simulink model "CONTROL_01"  (R2018b)
settings: Solver=FixedStepAuto  StartTime=0.0  StopTime=30  FixedStep=0.01  RelTol=1e-3
model workspace: external: MATLAB File D:\OneDrive\STUDY\RIC LAB\PROJECT 6DOF\CODE\CODE 6DOF\07_CONTROL\CONTROL_02\ROBOT_DataFile.m (data not in the file)
undefined symbols (not defined in the file or in its folder): smiData, X, Y, Z
libraries: sm_lib x35, nesl_utility x7
(part 1 of 185)
settings Model: Creator=TMP  LastModifiedBy=TMP
settings DataIOCC: SaveTime=off
settings DebuggingCC: AlgebraicLoopMsg=none

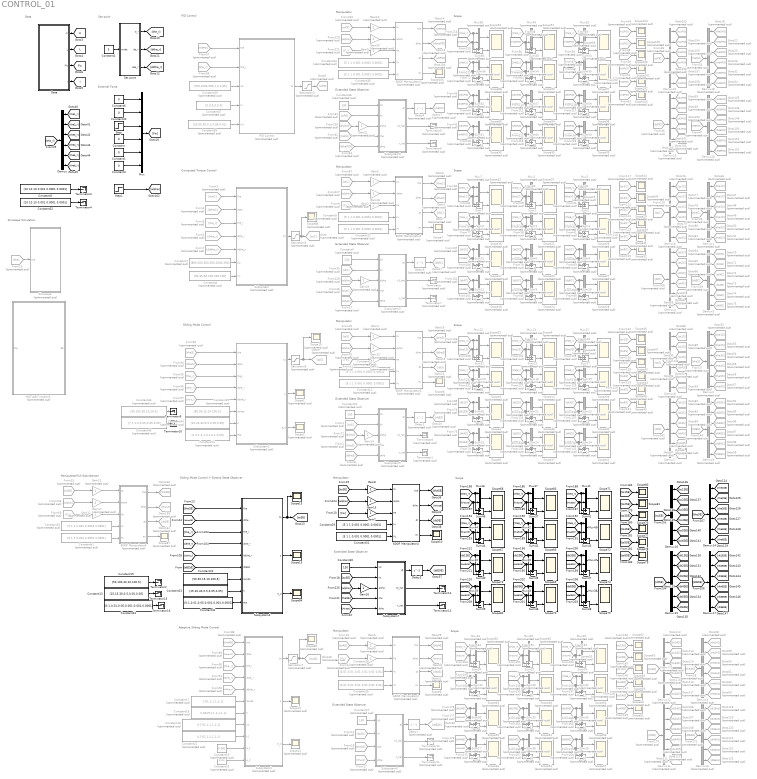
== system CONTROL_01 ==
  note: Extended State Observer
  note: Set point
  note: Simscape Simulation
  note: Data
  note: External Force
  note: Computed Torque Control
  note: Manipulator
  note: Sliding Mode Control
  note: Adaptive Sliding Mode Control
  note: Sliding Mode Control + Extend State Observer
  note: Extended State Observer
  note: Manipulator
  note: Extended State Observer
  note: Manipulator
  note: Extended State Observer
  note: Manipulator
  note: Scope
  note: Scope
  note: Scope
  note: Scope
  note: Extended State Observer
  note: PID Control
  note: Manipulator
  note: Scope
  note: Manipulator(full disturbance)
  6DOF Manipulator1 : Subsystem  Commented=on
  6DOF Manipulator2 : Subsystem  Commented=on
  6DOF Manipulator3 : Subsystem  Commented=on
  6DOF Manipulator4 : Subsystem
  6DOF Manipulator5 : Subsystem  Commented=on
  6DOF Manipulator6 : Subsystem  Commented=on
  Constant{,1,3,6,40} (5 alike) : Constant  Value=0
  Constant{9..12,33..35,41} (8 alike) : Constant  Commented=on  Value=[5 1 1 0.001 0.0001 0.0001]
  Constant13 : Constant  Value=[15,15,30,0.5,0.05,0.05]
  Constant14 : Constant  Commented=on  Value=[1.5,1.2,1,0.1,0.1,0.05]
  Constant15 : Constant  Value=[50,100,30,10,100,5]
  Constant16 : Constant  Commented=on  Value=0.001*[1,1,1,1,1,1]
  Constant17 : Constant  Commented=on  Value=1*[1,1,1,1,1,1]
  Constant18 : Constant  Commented=on  Value=0.1*[1,1,1,1,1,1]
  Constant19 : Constant  Commented=on  Value=0.001
  Constant2 : Constant  Value=3
  Constant20 : Constant  Commented=on  Value=0.01
  Constant21 : Constant  Commented=on  Value=0.1*[1,1,1,1,1,1]
  Constant22 : Constant  Commented=on  Value=130
  Constant23 : Constant  Value=[15,20,30,0.5,0.05,0.05]
  Constant24 : Constant  Value=[50,50,15,10,100,5]
  Constant25 : Constant  Commented=on  Value=[50,50,15,10,100,5]
  Constant26 : Constant  Commented=on  Value=[0.01 0.01 0.01 0.01 0.01 0.01]
  Constant27 : Constant  Commented=on  Value=100
  Constant28 : Constant  Commented=on  Value=[0.01 0.01 0.01 0.01 0.01 0.01]
  Constant29 : Constant  Value=[5 1 1 0.001 0.0001 0.0001]
  Constant30 : Constant  Value=130
  Constant31 : Constant  Value=[5 1 1 0.001 0.0001 0.0001]
  Constant32 : Constant  Value=[10 10 10 0.001 0.0001 0.0001]
  Constant36 : Constant  Commented=on  Value=130
  Constant37 : Constant  Commented=on  Value=[0,0,0,0,0,0]
  Constant38 : Constant  Commented=on  Value=[20,50,30,0.1,0.06,0.01]
  Constant39 : Constant  Commented=on  Value=[700,1200,500,1,2,0.05]
  Constant4 : Constant  Commented=on  Value=130
  Constant42 : Constant  Value=[0.1,0.01,0.05,0.001,0.001,0.0001]
  Constant43 : Constant  Value=[0.1,0.01,0.05,0.001,0.001,0.0001]
  Constant44 : Constant  Commented=on  Value=[15,20,30,0.5,0.05,0.05]
  Constant45 : Constant  Commented=on  Value=[7,7,1.2,0.05,0.05,0.05]
  Constant46 : Constant  Commented=on  Value=[50,100,30,10,10,5]
  Constant5 : Constant  Value=[10 10 10 0.001 0.0001 0.0001]
  Constant7 : Constant  Commented=on  Value=[800,200,500,500,2000,300]
  Constant8 : Constant  Commented=on  Value=[50,35,50,100,200,100]
  Data : MATLAB Function  TreatAsAtomicUnit=on
  Delay{1..2,4..5} (4 alike) : Delay  Commented=on  DelayLength=1
  Delay3 : Delay  DelayLength=1
  Demux{,14..17} (5 alike) : Demux  Outputs=6
  Demux{1..9,11..13,18..21} (16 alike) : Demux  Commented=on  Outputs=6
  From1 : From  Commented=on  GotoTag=toS
  From10 : From  Commented=on  GotoTag=toS
  From100 : From  Commented=on  GotoTag=dt6C
  From101 : From  Commented=on  GotoTag=dt4EC
  From102 : From  Commented=on  GotoTag=dt4C
  From106 : From  Commented=on  GotoTag=dt1EC
  From107 : From  Commented=on  GotoTag=dt1C
  From108 : From  Commented=on  GotoTag=dtC
  From109 : From  Commented=on  GotoTag=dtEC
  From{9,11,14,69,221} (5 alike) : From  Commented=on  GotoTag=Fe
  From110 : From  Commented=on  GotoTag=toC
  From111 : From  Commented=on  GotoTag=to2C
  From112 : From  Commented=on  GotoTag=to3C
  From113 : From  Commented=on  GotoTag=to4C
  From114 : From  Commented=on  GotoTag=to5C
  From115 : From  Commented=on  GotoTag=to6C
  From116 : From  Commented=on  GotoTag=to2S
  From117 : From  Commented=on  GotoTag=to1C
  From118 : From  Commented=on  GotoTag=to3S
  From119 : From  Commented=on  GotoTag=to4S
  From12 : From  Commented=on  GotoTag=toAS
  From120 : From  Commented=on  GotoTag=to5S
  From121 : From  Commented=on  GotoTag=to6S
  From122 : From  Commented=on  GotoTag=to1S
  From123 : From  Commented=on  GotoTag=the2S
  From{30,58,124,152} (4 alike) : From  Commented=on  GotoTag=the2_r
  From125 : From  Commented=on  GotoTag=the3S
  From{32,60,126,154} (4 alike) : From  Commented=on  GotoTag=the3_r
  From127 : From  Commented=on  GotoTag=the5S
  From{39,65,128,156} (4 alike) : From  Commented=on  GotoTag=the5_r
  From129 : From  Commented=on  GotoTag=the6S
  From13 : From  Commented=on  GotoTag=toAS
  From{42,68,130,158} (4 alike) : From  Commented=on  GotoTag=the6_r
  From131 : From  Commented=on  GotoTag=the4S
  From{78,132,160,173} (4 alike) : From  Commented=on  GotoTag=the4_r
  From133 : From  Commented=on  GotoTag=dt2ES
  From134 : From  Commented=on  GotoTag=dt2S
  From135 : From  Commented=on  GotoTag=the1S
  From{82,136,164,216} (4 alike) : From  Commented=on  GotoTag=the1_r
  From137 : From  Commented=on  GotoTag=dt3ES
  From138 : From  Commented=on  GotoTag=dt3S
  From139 : From  Commented=on  GotoTag=dt5ES
  From140 : From  Commented=on  GotoTag=dt5S
  From141 : From  Commented=on  GotoTag=dt6ES
  From142 : From  Commented=on  GotoTag=dtS
  From143 : From  Commented=on  GotoTag=toS
  From144 : From  Commented=on  GotoTag=dtES
  From145 : From  Commented=on  GotoTag=to2AS
  From146 : From  Commented=on  GotoTag=to3AS
  From147 : From  Commented=on  GotoTag=to4AS
  From148 : From  Commented=on  GotoTag=to5AS
  From149 : From  Commented=on  GotoTag=to6AS
  From15 : From  Commented=on  GotoTag=the  TagVisibility=global
  From150 : From  Commented=on  GotoTag=to1AS
  From151 : From  Commented=on  GotoTag=the2AS
  From153 : From  Commented=on  GotoTag=the3AS
  From155 : From  Commented=on  GotoTag=the5AS
  From157 : From  Commented=on  GotoTag=the6AS
  From159 : From  Commented=on  GotoTag=the4AS
  From16 : From  Commented=on  GotoTag=theAS
  From161 : From  Commented=on  GotoTag=dt2EAS
  From162 : From  Commented=on  GotoTag=dt2AS
  From163 : From  Commented=on  GotoTag=the1AS
  From165 : From  Commented=on  GotoTag=dt3EAS
  From166 : From  Commented=on  GotoTag=dt3AS
  From167 : From  Commented=on  GotoTag=dt5EAS
  From168 : From  Commented=on  GotoTag=dt5AS
  From169 : From  Commented=on  GotoTag=dt6EAS
  From17 : From  Commented=on  GotoTag=dtheAS
  From170 : From  Commented=on  GotoTag=dtAS
  From171 : From  Commented=on  GotoTag=toAS
  From172 : From  Commented=on  GotoTag=dtEAS
  From174 : From  Commented=on  GotoTag=dt6AS
  From175 : From  Commented=on  GotoTag=dt4EAS
  From176 : From  Commented=on  GotoTag=dt4AS
  From177 : From  Commented=on  GotoTag=dt1EAS
  From178 : From  Commented=on  GotoTag=dt1AS
  From2 : From  Commented=on  GotoTag=theS
  From213 : From  Commented=on  GotoTag=dt2EPID
  From214 : From  Commented=on  GotoTag=dt2PID
  From215 : From  Commented=on  GotoTag=the1PID
  From217 : From  Commented=on  GotoTag=dt3EPID
  From218 : From  Commented=on  GotoTag=dt3PID
  From219 : From  Commented=on  GotoTag=dt5EPID
  From220 : From  Commented=on  GotoTag=toPID  TagVisibility=global
  From222 : From  Commented=on  GotoTag=dt5PID
  From223 : From  Commented=on  GotoTag=dt6EPID
  From{70..71,226..230} (7 alike) : From  Commented=on  GotoTag=alpha
  From26 : From  Commented=on  GotoTag=theC
  From27 : From  Commented=on  GotoTag=theS
  From28 : From  Commented=on  GotoTag=theAS
  From29 : From  Commented=on  GotoTag=the2C
  From3 : From  Commented=on  GotoTag=theC
  From31 : From  Commented=on  GotoTag=the3C
  From33 : From  Commented=on  GotoTag=toSE
  From34 : From  Commented=on  GotoTag=dt6PID
  From35 : From  Commented=on  GotoTag=toC
  From36 : From  Commented=on  GotoTag=theC
  From37 : From  Commented=on  GotoTag=dtheC
  From38 : From  Commented=on  GotoTag=the5C
  From4 : From  Commented=on  GotoTag=dtheC
  From40 : From  Commented=on  GotoTag=dt4EPID
  From41 : From  Commented=on  GotoTag=the6C
  From43 : From  Commented=on  GotoTag=dt4PID
  From44 : From  Commented=on  GotoTag=dt1EPID
  From45 : From  Commented=on  GotoTag=dt1PID
  From46 : From  Commented=on  GotoTag=dtPID
  From47 : From  Commented=on  GotoTag=dtEPID
  From48 : From  Commented=on  GotoTag=toPID  TagVisibility=global
  From49 : From  Commented=on  GotoTag=to2PID
  From{5,66,90,95} (4 alike) : From  Commented=on  GotoTag=the_r
  From50 : From  Commented=on  GotoTag=to3PID
  From51 : From  Commented=on  GotoTag=to4PID
  From52 : From  Commented=on  GotoTag=to5PID
  From53 : From  Commented=on  GotoTag=to6PID
  From54 : From  Commented=on  GotoTag=to1PID
  From55 : From  Commented=on  GotoTag=thePID
  From56 : From  Commented=on  GotoTag=the2PID
  From57 : From  Commented=on  GotoTag=thePID
  From59 : From  Commented=on  GotoTag=the3PID
  From6 : From  Commented=on  GotoTag=dthe_r
  From61 : From  Commented=on  GotoTag=toPID  TagVisibility=global
  From62 : From  Commented=on  GotoTag=thePID
  From63 : From  Commented=on  GotoTag=dthePID
  From64 : From  Commented=on  GotoTag=the5PID
  From67 : From  Commented=on  GotoTag=the6PID
  From7 : From  Commented=on  GotoTag=ddthe_r
  From72 : From  Commented=on  GotoTag=the4PID
  From73 : From  Commented=on  GotoTag=dt6S
  From74 : From  Commented=on  GotoTag=dt4ES
  From75 : From  Commented=on  GotoTag=dt4S
  From76 : From  Commented=on  GotoTag=dt1ES
  From77 : From  Commented=on  GotoTag=the4C
  From79 : From  Commented=on  GotoTag=dt2EC
  From8 : From  Commented=on  GotoTag=dtheS
  From80 : From  Commented=on  GotoTag=dt2C
  From81 : From  Commented=on  GotoTag=the1C
  From83 : From  Commented=on  GotoTag=dt3EC
  From84 : From  Commented=on  GotoTag=dt3C
  From85 : From  Commented=on  GotoTag=dt1S
  From86 : From  Commented=on  GotoTag=dt5EC
  From87 : From  Commented=on  GotoTag=toC
  From88 : From  Commented=on  GotoTag=theAS
  From89 : From  Commented=on  GotoTag=dtheAS
  From91 : From  Commented=on  GotoTag=dthe_r
  From92 : From  Commented=on  GotoTag=ddthe_r
  From93 : From  Commented=on  GotoTag=theS
  From94 : From  Commented=on  GotoTag=dtheS
  From96 : From  Commented=on  GotoTag=dthe_r
  From97 : From  Commented=on  GotoTag=ddthe_r
  From98 : From  Commented=on  GotoTag=dt5C
  From99 : From  Commented=on  GotoTag=dt6EC
  Gain{1..6,9..14,17..21} (17 alike) : Gain  Commented=on
  Gain{7..8,15..16} (4 alike) : Gain
  Goto : Goto  Commented=on  GotoTag=toC
  Goto1 : Goto  Commented=on  GotoTag=dtheC
  Goto100 : Goto  Commented=on  GotoTag=dt3PID
  Goto101 : Goto  Commented=on  GotoTag=dt4PID
  Goto102 : Goto  Commented=on  GotoTag=dt5PID
  Goto103 : Goto  Commented=on  GotoTag=dt6PID
  Goto104 : Goto  Commented=on  GotoTag=dtPID
  Goto105 : Goto  Commented=on  GotoTag=dt1EPID
  Goto106 : Goto  Commented=on  GotoTag=dt1AS
  Goto107 : Goto  Commented=on  GotoTag=dt2AS
  Goto108 : Goto  Commented=on  GotoTag=dt3AS
  Goto109 : Goto  Commented=on  GotoTag=dt4AS
  Goto110 : Goto  Commented=on  GotoTag=dt5AS
  Goto111 : Goto  Commented=on  GotoTag=dt6AS
  Goto112 : Goto  Commented=on  GotoTag=to1AS
  Goto113 : Goto  Commented=on  GotoTag=to2AS
  Goto114 : Goto  Commented=on  GotoTag=to3AS
  Goto115 : Goto  Commented=on  GotoTag=to4AS
  Goto116 : Goto  Commented=on  GotoTag=to5AS
  Goto117 : Goto  Commented=on  GotoTag=to6AS
  Goto118 : Goto  Commented=on  GotoTag=dt1EAS
  Goto119 : Goto  Commented=on  GotoTag=dt2EAS
  Goto120 : Goto  Commented=on  GotoTag=dt3EAS
  Goto121 : Goto  Commented=on  GotoTag=dt4EAS
  Goto122 : Goto  Commented=on  GotoTag=dt5EAS
  Goto123 : Goto  Commented=on  GotoTag=dt6EAS
  Goto13 : Goto  Commented=on  GotoTag=dthePID
  Goto14 : Goto  Commented=on  GotoTag=thePID
  Goto148 : Goto  Commented=on  GotoTag=dt2EPID
  Goto149 : Goto  Commented=on  GotoTag=dt3EPID
  Goto15 : Goto  Commented=on  GotoTag=dtheS
  Goto150 : Goto  Commented=on  GotoTag=dt4EPID
  Goto151 : Goto  Commented=on  GotoTag=dt5EPID
  Goto152 : Goto  Commented=on  GotoTag=dt6EPID
  Goto153 : Goto  Commented=on  GotoTag=to1PID
  Goto154 : Goto  Commented=on  GotoTag=to2PID
  Goto155 : Goto  Commented=on  GotoTag=to3PID
  Goto156 : Goto  Commented=on  GotoTag=to4PID
  Goto157 : Goto  Commented=on  GotoTag=to5PID
  Goto158 : Goto  Commented=on  GotoTag=to6PID
  Goto159 : Goto  Commented=on  GotoTag=dtheSE
  Goto160 : Goto  Commented=on  GotoTag=theSE
  Goto161 : Goto  Commented=on  GotoTag=dtSE
  Goto17 : Goto  Commented=on  GotoTag=dtEPID
  Goto18 : Goto  Commented=on  GotoTag=the1PID
  Goto19 : Goto  Commented=on  GotoTag=theS
  Goto2 : Goto  Commented=on  GotoTag=theC
  Goto20 : Goto  Commented=on  GotoTag=dtES
  Goto21 : Goto  Commented=on  GotoTag=dtS
  Goto22 : Goto  Commented=on  GotoTag=the2PID
  Goto24 : Goto  Commented=on  GotoTag=dtheAS
  Goto25 : Goto  Commented=on  GotoTag=the3PID
  Goto26 : Goto  Commented=on  GotoTag=the4PID
  Goto27 : Goto  Commented=on  GotoTag=dtEC
  Goto28 : Goto  Commented=on  GotoTag=toAS
  Goto29 : Goto  Commented=on  GotoTag=theAS
  Goto30 : Goto  Commented=on  GotoTag=dtEAS
  Goto31 : Goto  Commented=on  GotoTag=dtAS
  Goto32 : Goto  Commented=on  GotoTag=the5PID
  Goto34 : Goto  Commented=on  GotoTag=the6PID
  Goto35 : Goto  Commented=on  GotoTag=dt1PID
  Goto39 : Goto  Commented=on  GotoTag=dt2PID
  Goto46 : Goto  Commented=on  GotoTag=the1C
  Goto47 : Goto  Commented=on  GotoTag=the2C
  Goto48 : Goto  Commented=on  GotoTag=the3C
  Goto49 : Goto  Commented=on  GotoTag=the4C
  Goto50 : Goto  Commented=on  GotoTag=the5C
  Goto51 : Goto  Commented=on  GotoTag=the6C
  Goto52 : Goto  Commented=on  GotoTag=the1S
  Goto53 : Goto  Commented=on  GotoTag=the2S
  Goto54 : Goto  Commented=on  GotoTag=the3S
  Goto55 : Goto  Commented=on  GotoTag=the4S
  Goto56 : Goto  Commented=on  GotoTag=the5S
  Goto57 : Goto  Commented=on  GotoTag=the6S
  Goto58 : Goto  Commented=on  GotoTag=the1AS
  Goto59 : Goto  Commented=on  GotoTag=the2AS
  Goto60 : Goto  Commented=on  GotoTag=the3AS
  Goto61 : Goto  Commented=on  GotoTag=the4AS
  Goto62 : Goto  Commented=on  GotoTag=the5AS
  Goto63 : Goto  Commented=on  GotoTag=the6AS
  Goto64 : Goto  Commented=on  GotoTag=dt1C
  Goto65 : Goto  Commented=on  GotoTag=dt2C
  Goto66 : Goto  Commented=on  GotoTag=dt3C
  Goto67 : Goto  Commented=on  GotoTag=dt4C
  Goto68 : Goto  Commented=on  GotoTag=dt5C
  Goto69 : Goto  Commented=on  GotoTag=dt6C
  Goto7 : Goto  Commented=on  GotoTag=dtC
  Goto70 : Goto  Commented=on  GotoTag=dt1EC
  Goto71 : Goto  Commented=on  GotoTag=dt2EC
  Goto72 : Goto  Commented=on  GotoTag=dt3EC
  Goto73 : Goto  Commented=on  GotoTag=dt4EC
  Goto74 : Goto  Commented=on  GotoTag=dt5EC
  Goto75 : Goto  Commented=on  GotoTag=dt6EC
  Goto76 : Goto  Commented=on  GotoTag=to1C
  Goto77 : Goto  Commented=on  GotoTag=to2C
  Goto78 : Goto  Commented=on  GotoTag=to3C
  Goto79 : Goto  Commented=on  GotoTag=to4C
  Goto8 : Goto  Commented=on  GotoTag=toPID  TagVisibility=global
  Goto80 : Goto  Commented=on  GotoTag=to5C
  Goto81 : Goto  Commented=on  GotoTag=to6C
  Goto82 : Goto  Commented=on  GotoTag=dt1S
  Goto83 : Goto  Commented=on  GotoTag=dt2S
  Goto84 : Goto  Commented=on  GotoTag=dt3S
  Goto85 : Goto  Commented=on  GotoTag=dt4S
  Goto86 : Goto  Commented=on  GotoTag=dt5S
  Goto87 : Goto  Commented=on  GotoTag=dt6S
  Goto88 : Goto  Commented=on  GotoTag=to1S
  Goto89 : Goto  Commented=on  GotoTag=to2S
  Goto9 : Goto  Commented=on  GotoTag=toS
  Goto90 : Goto  Commented=on  GotoTag=to3S
  Goto91 : Goto  Commented=on  GotoTag=to4S
  Goto92 : Goto  Commented=on  GotoTag=to5S
  Goto93 : Goto  Commented=on  GotoTag=to6S
  Goto94 : Goto  Commented=on  GotoTag=dt1ES
  Goto95 : Goto  Commented=on  GotoTag=dt2ES
  Goto96 : Goto  Commented=on  GotoTag=dt3ES
  Goto97 : Goto  Commented=on  GotoTag=dt4ES
  Goto98 : Goto  Commented=on  GotoTag=dt5ES
  Goto99 : Goto  Commented=on  GotoTag=dt6ES
  MATLAB Function3 : MATLAB Function  Commented=on  TreatAsAtomicUnit=on
  Mux : Mux  Inputs=6
  Mux{1..36,49..60} (48 alike) : Mux  Commented=on  Inputs=2
  Mux{37..48} (12 alike) : Mux  Inputs=2
  PID Control : Subsystem  Commented=on
  Saturation{3,5..7} (4 alike) : Saturate  Commented=on  UpperLimit=500  LowerLimit=-500
  Scope{1..2,7..9,11..12,19,29..32,34..35,42..47,58..63,85..87,100..106} (36 alike) : Scope  Commented=on
  Scope{10,13,15,76..81,84} (10 alike) : Scope
  Scope{3..6,14,16..18,20..28,33,36..41,48..57,64..65,88..99} (48 alike) : Scope  Commented=on  NumInputPorts=2
  Scope{66..75,82..83} (12 alike) : Scope  NumInputPorts=2
  Set point : Subsystem
  Simscape : Subsystem  Commented=on
  Step : Step  Time=10  After=20  SampleTime=0
  Step1 : Step  Time=20  Before=1  After=0.8  SampleTime=0
  Subsystem : Subsystem  Commented=on
  Subsystem1 : Subsystem  Commented=on
  Subsystem2 : Subsystem  Commented=on
  Subsystem3 : Subsystem  Commented=on
  Subsystem4 : Subsystem
  Subsystem5 : Subsystem  Commented=on
  Subsystem6 : Subsystem  Commented=on
  Subsystem7 : Subsystem
  Subsystem9 : Subsystem  Commented=on
  Sum{1..36,49..60} (48 alike) : Sum  Commented=on  Inputs=+-
  Sum{37..48} (12 alike) : Sum  Inputs=+-
  Terminator{,1,5..8,11..12} (8 alike) : Terminator  Commented=on
  Terminator{2..4,9..10,13..16} (9 alike) : Terminator
  tag scope: I=global, L=global, Pic=global, m=global
  wires:
  Set point/3(dde_r) -> [ddthe_r]
  Set point/1(e_r) -> [the_r]
  Constant2/1 -> Set point/1(mode)
  Set point/2(de_r) -> [dthe_r]
  Data/1(m) -> [m]
  Data/2(L) -> [L]
  Data/3(Pic) -> [Pic]
  Data/4(I) -> [I]
  From15/1 -> Simscape/1(the)
  Constant1/1 -> Mux/5
  Mux/1 -> [Fe]
  Constant3/1 -> Mux/6
  Constant/1 -> Mux/4
  Subsystem/1(to) -> Saturation5/1
  From3/1 -> Subsystem/1(the)
  From4/1 -> Subsystem/2(dthe)
  From5/1 -> Subsystem/3(the_r)
  From6/1 -> Subsystem/4(dthe_r)
  From7/1 -> Subsystem/5(ddthe_r)
  Saturation5/1 -> Goto/1, Scope86/1
  From87/1 -> Gain3/1
  6DOF Manipulator1/4(ex) -> Scope7/1
  6DOF Manipulator1/2(dthe) -> Goto1/1
  Gain3/1 -> 6DOF Manipulator1/1(to)
  Gain2/1 -> 6DOF Manipulator1/3(Fe)
  6DOF Manipulator1/3(dt) -> Goto7/1
  From9/1 -> Gain2/1
  Constant8/1 -> Subsystem/7(Kv)
  Constant7/1 -> Subsystem/6(Kp)
  Constant9/1 -> 6DOF Manipulator1/4(Fv)
  Constant12/1 -> 6DOF Manipulator1/5(Fc)
  Subsystem1/1(to) -> Saturation6/1
  Saturation6/1 -> Scope19/1, Goto9/1
  From93/1 -> Subsystem1/1(the)
  From94/1 -> Subsystem1/2(dthe)
  From95/1 -> Subsystem1/3(the_r)
  From96/1 -> Subsystem1/4(dthe_r)
  From97/1 -> Subsystem1/5(ddthe_r)
  Constant14/1 -> Subsystem1/8(eta)
  Constant44/1 -> Subsystem1/7(K)
  Constant25/1 -> Subsystem1/6(lamda)
  Subsystem1/2(s) -> Scope1/1
  Subsystem1/3(e_d) -> Scope2/1
  Constant18/1 -> Subsystem2/8(k1)
  From92/1 -> Subsystem2/5(ddthe_r)
  From91/1 -> Subsystem2/4(dthe_r)
  Subsystem2/1(to) -> Saturation7/1
  From88/1 -> Subsystem2/1(the)
  Constant16/1 -> Subsystem2/7(K)
  From90/1 -> Subsystem2/3(the_r)
  Saturation7/1 -> Scope85/1, Goto28/1
  Constant17/1 -> Subsystem2/6(lamda)
  From89/1 -> Subsystem2/2(dthe)
  Constant19/1 -> Subsystem2/10(e_1)
  Constant20/1 -> Subsystem2/11(e_2)
  Constant21/1 -> Subsystem2/9(k2)
  6DOF Manipulator1/1(the) -> Goto2/1
  Constant4/1 -> Subsystem3/1(k0)
  From35/1 -> Subsystem3/2(to)
  From36/1 -> Subsystem3/4(the)
  Subsystem3/2(x3_hat) -> Terminator/1
  Subsystem3/3(x_hat) -> Terminator7/1
  From37/1 -> Subsystem3/5(dthe)
  [dthe_r] -> Subsystem4/4(dthe_r)
  Constant42/1 -> Subsystem4/9(eta)
  Subsystem4/3(e_d) -> Scope84/1
  Subsystem4/2(s) -> Scope13/1
  Constant23/1 -> Subsystem4/8(K)
  [the_r] -> Subsystem4/3(the_r)
  Constant24/1 -> Subsystem4/7(lamda)
  [ddthe_r] -> Subsystem4/5(ddthe_r)
  Subsystem4/1(to) -> [toSE], Scope15/1
  From8/1 -> Subsystem5/5(dthe)
  Subsystem5/3(x_hat) -> Terminator1/1
  Subsystem5/2(x3_hat) -> Terminator8/1
  From2/1 -> Subsystem5/4(the)
  From1/1 -> Subsystem5/2(to)
  Constant22/1 -> Subsystem5/1(k0)
  Subsystem5/1("dt ") -> Delay2/1
  6DOF Manipulator2/1(the) -> Goto19/1
  From11/1 -> Gain1/1
  6DOF Manipulator2/3(dt) -> Goto21/1
  Gain1/1 -> 6DOF Manipulator2/3(Fe)
  Gain4/1 -> 6DOF Manipulator2/1(to)
  6DOF Manipulator2/2(dthe) -> Goto15/1
  6DOF Manipulator2/4(ex) -> Scope8/1
  From10/1 -> Gain4/1
  From13/1 -> Gain6/1
  6DOF Manipulator3/4(ex) -> Scope9/1
  6DOF Manipulator3/2(dthe) -> Goto24/1
  Gain6/1 -> 6DOF Manipulator3/1(to)
  Gain5/1 -> 6DOF Manipulator3/2(Fe)
  6DOF Manipulator3/3(dt) -> Goto31/1
  From14/1 -> Gain5/1
  Constant28/1 -> 6DOF Manipulator3/3(Fv)
  Constant26/1 -> 6DOF Manipulator3/4(Fc)
  6DOF Manipulator3/1(the) -> Goto29/1
  Subsystem6/1("dt ") -> Delay1/1
  Constant27/1 -> Subsystem6/1(k0)
  From12/1 -> Subsystem6/2(to)
  From16/1 -> Subsystem6/3(the)
  Subsystem6/2(x3_hat) -> Terminator12/1
  Subsystem6/3(x_hat) -> Terminator11/1
  From17/1 -> Subsystem6/4(dthe)
  Subsystem7/3(x_hat) -> Terminator13/1
  Subsystem7/2(x3_hat) -> Terminator14/1
  Constant30/1 -> Subsystem7/1(k0)
  Constant31/1 -> 6DOF Manipulator4/5(Fc)
  Constant29/1 -> 6DOF Manipulator4/4(Fv)
  [Fe] -> Gain7/1
  6DOF Manipulator4/3(dt) -> [dtSE]
  Gain7/1 -> 6DOF Manipulator4/3(Fe)
  Gain8/1 -> 6DOF Manipulator4/1(to)
  6DOF Manipulator4/2(dthe) -> [dtheSE]
  6DOF Manipulator4/4(ex) -> Scope10/1
  [toSE] -> Gain8/1
  [theSE] -> Subsystem4/1(the)
  [dtheSE] -> Subsystem4/2(dthe)
  [toSE] -> Subsystem7/2(to)
  [theSE] -> Subsystem7/4(the)
  [dtheSE] -> Subsystem7/5(dthe)
  Subsystem7/1("dt ") -> Delay3/1
  6DOF Manipulator4/1(the) -> [theSE]
  [dtESE] -> Subsystem4/6(dtESO)
  [the_r] -> Demux/1
  Demux/1 -> [the1_r]
  Demux/2 -> [the2_r]
  Demux/3 -> [the3_r]
  Demux/6 -> [the6_r]
  Demux/5 -> [the5_r]
  Demux/4 -> [the4_r]
  Demux1/4 -> Goto49/1
  Demux1/5 -> Goto50/1
  Demux1/6 -> Goto51/1
  Demux1/3 -> Goto48/1
  Demux1/2 -> Goto47/1
  Demux1/1 -> Goto46/1
  From26/1 -> Demux1/1
  From28/1 -> Demux3/1
  Demux3/1 -> Goto58/1
  Demux3/2 -> Goto59/1
  Demux3/3 -> Goto60/1
  Demux3/6 -> Goto63/1
  Demux3/5 -> Goto62/1
  Demux3/4 -> Goto61/1
  Demux2/4 -> Goto55/1
  Demux2/5 -> Goto56/1
  Demux2/6 -> Goto57/1
  Demux2/3 -> Goto54/1
  Demux2/2 -> Goto53/1
  Demux2/1 -> Goto52/1
  From27/1 -> Demux2/1
  From82/1 -> Sum7/1, Mux7/1
  From81/1 -> Sum7/2, Mux7/2
  Sum7/1 -> Scope22/2
  Mux7/1 -> Scope22/1
  Mux1/1 -> Scope20/1
  Sum1/1 -> Scope20/2
  From29/1 -> Mux1/2, Sum1/2
  From30/1 -> Mux1/1, Sum1/1
  From32/1 -> Sum2/1, Mux2/1
  From31/1 -> Sum2/2, Mux2/2
  Sum2/1 -> Scope25/2
  Mux2/1 -> Scope25/1
  Mux4/1 -> Scope26/1
  Sum4/1 -> Scope26/2
  From41/1 -> Mux4/2, Sum4/2
  From42/1 -> Mux4/1, Sum4/1
  From39/1 -> Sum3/1, Mux3/1
  From38/1 -> Sum3/2, Mux3/2
  Sum3/1 -> Scope21/2
  Mux3/1 -> Scope21/1
  Mux5/1 -> Scope16/1
  Sum5/1 -> Scope16/2
  From77/1 -> Mux5/2, Sum5/2
  From78/1 -> Mux5/1, Sum5/1
  From102/1 -> Sum11/1, Mux11/1
  From101/1 -> Sum11/2, Mux11/2
  Sum11/1 -> Scope18/2
  Mux11/1 -> Scope18/1
  Mux9/1 -> Scope24/1
  Sum9/1 -> Scope24/2
  From86/1 -> Mux9/2, Sum9/2
  From98/1 -> Mux9/1, Sum9/1
  From100/1 -> Sum10/1, Mux10/1
  From99/1 -> Sum10/2, Mux10/2
  Sum10/1 -> Scope28/2
  Mux10/1 -> Scope28/1
  Mux8/1 -> Scope27/1
  Sum8/1 -> Scope27/2
  From83/1 -> Mux8/2, Sum8/2
  From84/1 -> Mux8/1, Sum8/1
  From80/1 -> Sum6/1, Mux6/1
  From79/1 -> Sum6/2, Mux6/2
  Sum6/1 -> Scope23/2
  Mux6/1 -> Scope23/1
  Mux12/1 -> Scope17/1
  Sum12/1 -> Scope17/2
  From106/1 -> Mux12/2, Sum12/2
  Demux4/4 -> Goto67/1
  Demux4/5 -> Goto68/1
  Demux4/6 -> Goto69/1
  Demux4/3 -> Goto66/1
  Demux4/2 -> Goto65/1
  Demux4/1 -> Goto64/1
  From109/1 -> Demux5/1
  Demux5/1 -> Goto70/1
  Demux5/2 -> Goto71/1
  Demux5/3 -> Goto72/1
  Demux5/6 -> Goto75/1
  Demux5/5 -> Goto74/1
  Demux5/4 -> Goto73/1
  From115/1 -> Scope32/1
  From112/1 -> Scope29/1
  From117/1 -> Scope34/1
  From110/1 -> Demux6/1
  Demux6/1 -> Goto76/1
  Demux6/2 -> Goto77/1
  Demux6/3 -> Goto78/1
  Demux6/6 -> Goto81/1
  Demux6/5 -> Goto80/1
  Demux6/4 -> Goto79/1
  From111/1 -> Scope35/1
  From113/1 -> Scope30/1
  From114/1 -> Scope31/1
  From120/1 -> Scope44/1
  From119/1 -> Scope43/1
  From116/1 -> Scope47/1
  From122/1 -> Scope46/1
  From118/1 -> Scope42/1
  From121/1 -> Scope45/1
  From85/1 -> Sum16/1, Mux16/1
  From76/1 -> Sum16/2, Mux16/2
  Sum16/1 -> Scope4/2
  Mux16/1 -> Scope4/1
  Mux21/1 -> Scope36/1
  Sum21/1 -> Scope36/2
  From133/1 -> Mux21/2, Sum21/2
  From134/1 -> Mux21/1, Sum21/1
  From138/1 -> Sum23/1, Mux23/1
  From137/1 -> Sum23/2, Mux23/2
  Sum23/1 -> Scope40/2
  Mux23/1 -> Scope40/1
  Mux14/1 -> Scope41/1
  Sum14/1 -> Scope41/2
  From141/1 -> Mux14/2, Sum14/2
  From73/1 -> Mux14/1, Sum14/1
  From140/1 -> Sum24/1, Mux24/1
  From139/1 -> Sum24/2, Mux24/2
  Sum24/1 -> Scope37/2
  Mux24/1 -> Scope37/1
  Mux15/1 -> Scope5/1
  Sum15/1 -> Scope5/2
  From74/1 -> Mux15/2, Sum15/2
  From75/1 -> Mux15/1, Sum15/1
  From132/1 -> Sum20/1, Mux20/1
  From131/1 -> Sum20/2, Mux20/2
  Sum20/1 -> Scope3/2
  Mux20/1 -> Scope3/1
  Mux18/1 -> Scope14/1
  Sum18/1 -> Scope14/2
  From127/1 -> Mux18/2, Sum18/2
  From128/1 -> Mux18/1, Sum18/1
  From130/1 -> Sum19/1, Mux19/1
  From129/1 -> Sum19/2, Mux19/2
  Sum19/1 -> Scope39/2
  Mux19/1 -> Scope39/1
  Mux17/1 -> Scope38/1
  Sum17/1 -> Scope38/2
  From125/1 -> Mux17/2, Sum17/2
  From126/1 -> Mux17/1, Sum17/1
  From124/1 -> Sum13/1, Mux13/1
  From123/1 -> Sum13/2, Mux13/2
  Sum13/1 -> Scope6/2
  Mux13/1 -> Scope6/1
  Mux22/1 -> Scope33/1
  Sum22/1 -> Scope33/2
  From135/1 -> Mux22/2, Sum22/2
  From136/1 -> Mux22/1, Sum22/1
  Demux8/4 -> Goto91/1
  Demux8/5 -> Goto92/1
  Demux8/6 -> Goto93/1
  Demux8/3 -> Goto90/1
  Demux8/2 -> Goto89/1
  Demux8/1 -> Goto88/1
  From143/1 -> Demux8/1
  From142/1 -> Demux7/1
  Demux7/1 -> Goto82/1
  Demux7/2 -> Goto83/1
  Demux7/3 -> Goto84/1
  Demux7/6 -> Goto87/1
  Demux7/5 -> Goto86/1
  Demux7/4 -> Goto85/1
  Demux9/4 -> Goto97/1
  Demux9/5 -> Goto98/1
  Demux9/6 -> Goto99/1
  Demux9/3 -> Goto96/1
  Demux9/2 -> Goto95/1
  Demux9/1 -> Goto94/1
  From144/1 -> Demux9/1
  From172/1 -> Demux13/1
  Demux13/1 -> Goto118/1
  Demux13/2 -> Goto119/1
  Demux13/3 -> Goto120/1
  Demux13/6 -> Goto123/1
  Demux13/5 -> Goto122/1
  Demux13/4 -> Goto121/1
  Demux11/4 -> Goto109/1
  Demux11/5 -> Goto110/1
  Demux11/6 -> Goto111/1
  Demux11/3 -> Goto108/1
  Demux11/2 -> Goto107/1
  Demux11/1 -> Goto106/1
  From170/1 -> Demux11/1
  From171/1 -> Demux12/1
  Demux12/1 -> Goto112/1
  Demux12/2 -> Goto113/1
  Demux12/3 -> Goto114/1
  Demux12/6 -> Goto117/1
  Demux12/5 -> Goto116/1
  Demux12/4 -> Goto115/1
  From164/1 -> Sum34/1, Mux34/1
  From163/1 -> Sum34/2, Mux34/2
  Sum34/1 -> Scope50/2
  Mux34/1 -> Scope50/1
  Mux25/1 -> Scope65/1
  Sum25/1 -> Scope65/2
  From151/1 -> Mux25/2, Sum25/2
  From152/1 -> Mux25/1, Sum25/1
  From154/1 -> Sum29/1, Mux29/1
  From153/1 -> Sum29/2, Mux29/2
  Sum29/1 -> Scope53/2
  Mux29/1 -> Scope53/1
  Mux31/1 -> Scope54/1
  Sum31/1 -> Scope54/2
  From157/1 -> Mux31/2, Sum31/2
  From158/1 -> Mux31/1, Sum31/1
  From156/1 -> Sum30/1, Mux30/1
  From155/1 -> Sum30/2, Mux30/2
  Sum30/1 -> Scope48/2
  Mux30/1 -> Scope48/1
  Mux32/1 -> Scope49/1
  Sum32/1 -> Scope49/2
  From159/1 -> Mux32/2, Sum32/2
  From160/1 -> Mux32/1, Sum32/1
  From176/1 -> Sum27/1, Mux27/1
  From175/1 -> Sum27/2, Mux27/2
  Sum27/1 -> Scope64/2
  Mux27/1 -> Scope64/1
  Mux36/1 -> Scope52/1
  Sum36/1 -> Scope52/2
  From167/1 -> Mux36/2, Sum36/2
  From168/1 -> Mux36/1, Sum36/1
  From174/1 -> Sum26/1, Mux26/1
  From169/1 -> Sum26/2, Mux26/2
  Sum26/1 -> Scope57/2
  Mux26/1 -> Scope57/1
  Mux35/1 -> Scope56/1
  Sum35/1 -> Scope56/2
  From165/1 -> Mux35/2, Sum35/2
  From166/1 -> Mux35/1, Sum35/1
  From162/1 -> Sum33/1, Mux33/1
  From161/1 -> Sum33/2, Mux33/2
  Sum33/1 -> Scope51/2
  Mux33/1 -> Scope51/1
  Mux28/1 -> Scope55/1
  Sum28/1 -> Scope55/2
  From177/1 -> Mux28/2, Sum28/2
  From178/1 -> Mux28/1, Sum28/1
  From149/1 -> Scope61/1
  From146/1 -> Scope58/1
  From150/1 -> Scope62/1
  From145/1 -> Scope63/1
  From147/1 -> Scope59/1
  From148/1 -> Scope60/1
  Demux14/4 -> [the4SE]
  Demux14/5 -> [the5SE]
  Demux14/6 -> [the6SE]
  Demux14/3 -> [the3SE]
  Demux14/2 -> [the2SE]
  Demux14/1 -> [the1SE]
  [theSE] -> Demux14/1
  [to5SE] -> Scope78/1
  [to4SE] -> Scope77/1
  [to2SE] -> Scope81/1
  [to1SE] -> Scope80/1
  [to3SE] -> Scope76/1
  [to6SE] -> Scope79/1
  [dt1SE] -> Sum40/1, Mux40/1
  [dt1ESE] -> Sum40/2, Mux40/2
  Sum40/1 -> Scope73/2
  Mux40/1 -> Scope73/1
  Mux45/1 -> Scope69/1
  Sum45/1 -> Scope69/2
  [dt2ESE] -> Mux45/2, Sum45/2
  [dt2SE] -> Mux45/1, Sum45/1
  [dt3SE] -> Sum47/1, Mux47/1
  [dt3ESE] -> Sum47/2, Mux47/2
  Sum47/1 -> Scope74/2
  Mux47/1 -> Scope74/1
  Mux38/1 -> Scope75/1
  Sum38/1 -> Scope75/2
  [dt6ESE] -> Mux38/2, Sum38/2
  [dt6SE] -> Mux38/1, Sum38/1
  [dt5SE] -> Sum48/1, Mux48/1
  [dt5ESE] -> Sum48/2, Mux48/2
  Sum48/1 -> Scope70/2
  Mux48/1 -> Scope70/1
  Mux39/1 -> Scope82/1
  Sum39/1 -> Scope82/2
  [dt4ESE] -> Mux39/2, Sum39/2
  [dt4SE] -> Mux39/1, Sum39/1
  [the4_r] -> Sum44/1, Mux44/1
  [the4SE] -> Sum44/2, Mux44/2
  Sum44/1 -> Scope67/2
  Mux44/1 -> Scope67/1
  Mux42/1 -> Scope66/1
  Sum42/1 -> Scope66/2
  [the5SE] -> Mux42/2, Sum42/2
  [the5_r] -> Mux42/1, Sum42/1
  [the6_r] -> Sum43/1, Mux43/1
  [the6SE] -> Sum43/2, Mux43/2
  Sum43/1 -> Scope72/2
  Mux43/1 -> Scope72/1
  Mux41/1 -> Scope71/1
  Sum41/1 -> Scope71/2
  [the3SE] -> Mux41/2, Sum41/2
  [the3_r] -> Mux41/1, Sum41/1
  [the2_r] -> Sum37/1, Mux37/1
  [the2SE] -> Sum37/2, Mux37/2
  Sum37/1 -> Scope83/2
  Mux37/1 -> Scope83/1
  Mux46/1 -> Scope68/1
  Sum46/1 -> Scope68/2
  [the1SE] -> Mux46/2, Sum46/2
  [the1_r] -> Mux46/1, Sum46/1
  Demux16/4 -> [to4SE]
  Demux16/5 -> [to5SE]
  Demux16/6 -> [to6SE]
  Demux16/3 -> [to3SE]
  Demux16/2 -> [to2SE]
  Demux16/1 -> [to1SE]
  [toSE] -> Demux16/1
  Demux15/1 -> [dt1SE]
  Demux15/2 -> [dt2SE]
  Demux15/3 -> [dt3SE]
  Demux15/6 -> [dt6SE]
  Demux15/5 -> [dt5SE]
  Demux15/4 -> [dt4SE]
  Demux17/4 -> [dt4ESE]
  Demux17/5 -> [dt5ESE]
  Demux17/6 -> [dt6ESE]
  Demux17/3 -> [dt3ESE]
  Demux17/2 -> [dt2ESE]
  Demux17/1 -> [dt1ESE]
  [dtESE] -> Demux17/1
  Subsystem2/3(e_d) -> Scope12/1
  Subsystem2/2(s) -> Scope11/1
  Delay2/1 -> Goto20/1
  Delay1/1 -> Goto30/1
  Delay3/1 -> [dtESE]
  Subsystem3/1("dt ") -> Delay5/1
  From107/1 -> Sum12/1, Mux12/1
  From108/1 -> Demux4/1
  Delay5/1 -> Goto27/1
  Constant10/1 -> 6DOF Manipulator2/4(Fv)
  Constant11/1 -> 6DOF Manipulator2/5(Fc)
  Constant5/1 -> Terminator3/1
  Constant32/1 -> Terminator4/1
  Delay4/1 -> Goto17/1
  From46/1 -> Demux19/1
  From45/1 -> Mux52/1, Sum52/1
  Subsystem9/1("dt ") -> Delay4/1
  From52/1 -> Scope102/1
  From51/1 -> Scope101/1
  From49/1 -> Scope105/1
  Demux21/4 -> Goto156/1
  Demux21/5 -> Goto157/1
  Demux21/6 -> Goto158/1
  Demux21/3 -> Goto155/1
  Demux21/2 -> Goto154/1
  Demux21/1 -> Goto153/1
  From48/1 -> Demux21/1
  From54/1 -> Scope104/1
  From50/1 -> Scope100/1
  From53/1 -> Scope103/1
  Demux20/4 -> Goto150/1
  Demux20/5 -> Goto151/1
  Demux20/6 -> Goto152/1
  Demux20/3 -> Goto149/1
  Demux20/2 -> Goto148/1
  Demux20/1 -> Goto105/1
  From47/1 -> Demux20/1
  Demux19/1 -> Goto35/1
  Demux19/2 -> Goto39/1
  Demux19/3 -> Goto100/1
  Demux19/6 -> Goto103/1
  Demux19/5 -> Goto102/1
  Demux19/4 -> Goto101/1
  From44/1 -> Sum52/2, Mux52/2
  Sum52/1 -> Scope89/2
  Mux52/1 -> Scope89/1
  Mux57/1 -> Scope94/1
  Sum57/1 -> Scope94/2
  From213/1 -> Mux57/2, Sum57/2
  From214/1 -> Mux57/1, Sum57/1
  From218/1 -> Sum59/1, Mux59/1
  From217/1 -> Sum59/2, Mux59/2
  Sum59/1 -> Scope98/2
  Mux59/1 -> Scope98/1
  Mux50/1 -> Scope99/1
  Sum50/1 -> Scope99/2
  From223/1 -> Mux50/2, Sum50/2
  From34/1 -> Mux50/1, Sum50/1
  From222/1 -> Sum60/1, Mux60/1
  From219/1 -> Sum60/2, Mux60/2
  Sum60/1 -> Scope95/2
  Mux60/1 -> Scope95/1
  Mux51/1 -> Scope90/1
  Sum51/1 -> Scope90/2
  From40/1 -> Mux51/2, Sum51/2
  From43/1 -> Mux51/1, Sum51/1
  From173/1 -> Sum56/1, Mux56/1
  From72/1 -> Sum56/2, Mux56/2
  Sum56/1 -> Scope88/2
  Mux56/1 -> Scope88/1
  Mux54/1 -> Scope92/1
  Sum54/1 -> Scope92/2
  From64/1 -> Mux54/2, Sum54/2
  From65/1 -> Mux54/1, Sum54/1
  From68/1 -> Sum55/1, Mux55/1
  From67/1 -> Mux55/2, Sum55/2
  Sum55/1 -> Scope97/2
  Mux55/1 -> Scope97/1
  Mux53/1 -> Scope96/1
  Sum53/1 -> Scope96/2
  From59/1 -> Mux53/2, Sum53/2
  From60/1 -> Mux53/1, Sum53/1
  From58/1 -> Sum49/1, Mux49/1
  From56/1 -> Sum49/2, Mux49/2
  Sum49/1 -> Scope91/2
  Mux49/1 -> Scope91/1
  Mux58/1 -> Scope93/1
  Sum58/1 -> Scope93/2
  From215/1 -> Mux58/2, Sum58/2
  From216/1 -> Mux58/1, Sum58/1
  From55/1 -> Demux18/1
  Demux18/1 -> Goto18/1
  Demux18/2 -> Goto22/1
  Demux18/3 -> Goto25/1
  Demux18/6 -> Goto34/1
  Demux18/5 -> Goto32/1
  Demux18/4 -> Goto26/1
  From63/1 -> Subsystem9/5(dthe)
  Subsystem9/3(x_hat) -> Terminator6/1
  Subsystem9/2(x3_hat) -> Terminator5/1
  From62/1 -> Subsystem9/4(the)
  From61/1 -> Subsystem9/2(to)
  Constant36/1 -> Subsystem9/1(k0)
  6DOF Manipulator5/1(the) -> Goto14/1
  From221/1 -> Gain9/1
  6DOF Manipulator5/3(dt) -> Goto104/1
  Gain9/1 -> 6DOF Manipulator5/3(Fe)
  Gain10/1 -> 6DOF Manipulator5/1(to)
  6DOF Manipulator5/2(dthe) -> Goto13/1
  6DOF Manipulator5/4(ex) -> Scope106/1
  From220/1 -> Gain10/1
  From57/1 -> PID Control/1(the)
  PID Control/1(to) -> Saturation3/1
  Saturation3/1 -> Goto8/1
  From66/1 -> PID Control/2(the_r)
  Constant39/1 -> PID Control/3(Kp)
  Constant38/1 -> PID Control/5(Kd)
  Constant37/1 -> PID Control/4(Ki)
  Constant34/1 -> 6DOF Manipulator5/4(Fv)
  Constant35/1 -> 6DOF Manipulator5/5(Fc)
  [dtSE] -> Demux15/1
  6DOF Manipulator6/1(the) -> Goto160/1
  From33/1 -> Gain12/1
  6DOF Manipulator6/4(ex) -> Scope87/1
  6DOF Manipulator6/2(dthe) -> Goto159/1
  Gain12/1 -> 6DOF Manipulator6/1(to)
  Gain11/1 -> 6DOF Manipulator6/3(Fe)
  6DOF Manipulator6/3(dt) -> Goto161/1
  From69/1 -> Gain11/1
  Constant33/1 -> 6DOF Manipulator6/4(Fv)
  Constant41/1 -> 6DOF Manipulator6/5(Fc)
  Constant46/1 -> Terminator9/1
  Constant45/1 -> Terminator10/1
  Step1/1 -> [alpha]
  From70/1 -> Gain13/1
  Gain13/1 -> 6DOF Manipulator2/2(alpha)
  Gain14/1 -> Subsystem5/3(alpha)
  From71/1 -> Gain14/1
  Gain15/1 -> 6DOF Manipulator4/2(alpha)
  [alpha] -> Gain15/1
  [alpha] -> Gain16/1
  Gain16/1 -> Subsystem7/3(alpha)
  Gain17/1 -> 6DOF Manipulator6/2(alpha)
  From226/1 -> Gain17/1
  Constant40/1 -> Mux/2
  Step/1 -> Mux/3
  Constant6/1 -> Mux/1
  From227/1 -> Gain18/1
  Gain18/1 -> 6DOF Manipulator1/2(alpha)
  From228/1 -> Gain19/1
  Gain19/1 -> Subsystem3/3(alpha)
  From229/1 -> Gain20/1
  Gain20/1 -> 6DOF Manipulator5/2(alpha)
  From230/1 -> Gain21/1
  Gain21/1 -> Subsystem9/3(alpha)
  Constant15/1 -> Terminator2/1
  Constant13/1 -> Terminator15/1
  Constant43/1 -> Terminator16/1

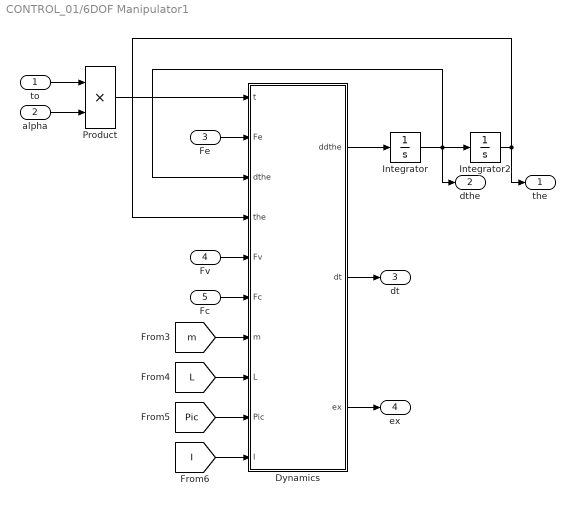
== system CONTROL_01/6DOF Manipulator1 ==
  to : Inport
  alpha : Inport  Port=2
  Fe : Inport  Port=3
  Fv : Inport  Port=4
  Fc : Inport  Port=5
  Dynamics : MATLAB Function  TreatAsAtomicUnit=on
  Integrator : Integrator  InitialCondition=[0;0;0;0;0;0]  UpperSaturationLimit=pi  LowerSaturationLimit=-pi
  Integrator2 : Integrator  InitialCondition=[0;0;0;0;0;0]  UpperSaturationLimit=[170;135;166;190;120;360]*pi/180  LowerSaturationLimit=-[170;100;119;190;120;360]*pi/180
  Product : Product
  the : Outport
  dthe : Outport  Port=2
  dt : Outport  Port=3
  ex : Outport  Port=4
  wires:
  Integrator2/1 -> Dynamics/4(the), the/1
  Dynamics/1(ddthe) -> Integrator/1
  Integrator/1 -> Dynamics/3(dthe), dthe/1, Integrator2/1
  Dynamics/2(dt) -> dt/1
  Fe/1 -> Dynamics/2(Fe)
  Dynamics/3(ex) -> ex/1
  [I] -> Dynamics/10(I)
  [Pic] -> Dynamics/9(Pic)
  [L] -> Dynamics/8(L)
  [m] -> Dynamics/7(m)
  Fv/1 -> Dynamics/5(Fv)
  Fc/1 -> Dynamics/6(Fc)
  alpha/1 -> Product/2
  to/1 -> Product/1
  Product/1 -> Dynamics/1(t)

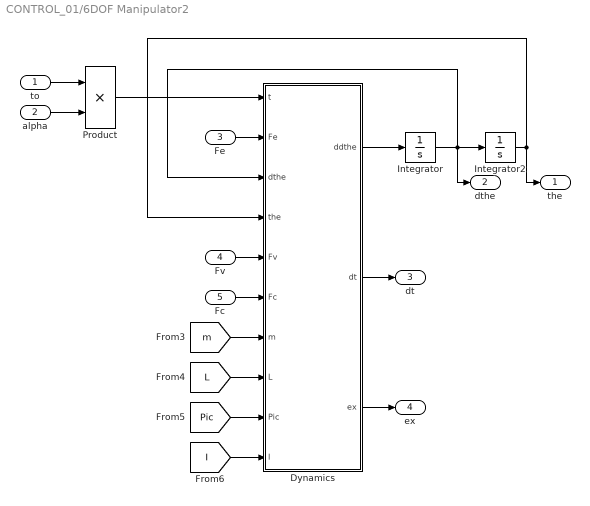
== system CONTROL_01/6DOF Manipulator2 ==
  to : Inport
  alpha : Inport  Port=2
  Fe : Inport  Port=3
  Fv : Inport  Port=4
  Fc : Inport  Port=5
  Dynamics : MATLAB Function  TreatAsAtomicUnit=on
  Integrator : Integrator  InitialCondition=[0;0;0;0;0;0]  UpperSaturationLimit=pi  LowerSaturationLimit=-pi
  Integrator2 : Integrator  InitialCondition=[0;0;0;0;0;0]  UpperSaturationLimit=[170;135;166;190;120;360]*pi/180  LowerSaturationLimit=-[170;100;119;190;120;360]*pi/180
  Product : Product
  the : Outport
  dthe : Outport  Port=2
  dt : Outport  Port=3
  ex : Outport  Port=4
  wires:
  Fc/1 -> Dynamics/6(Fc)
  Fv/1 -> Dynamics/5(Fv)
  [m] -> Dynamics/7(m)
  [L] -> Dynamics/8(L)
  [Pic] -> Dynamics/9(Pic)
  [I] -> Dynamics/10(I)
  Dynamics/3(ex) -> ex/1
  Fe/1 -> Dynamics/2(Fe)
  Dynamics/2(dt) -> dt/1
  Integrator/1 -> Integrator2/1, dthe/1, Dynamics/3(dthe)
  Dynamics/1(ddthe) -> Integrator/1
  Integrator2/1 -> the/1, Dynamics/4(the)
  alpha/1 -> Product/2
  to/1 -> Product/1
  Product/1 -> Dynamics/1(t)

== system CONTROL_01/6DOF Manipulator3 ==
  to : Inport
  Fe : Inport  Port=2
  Fv : Inport  Port=3
  Fc : Inport  Port=4
  Dynamics : MATLAB Function  TreatAsAtomicUnit=on
  Integrator : Integrator  InitialCondition=[0;0;0;0;0;0]  LimitOutput=on  UpperSaturationLimit=pi  LowerSaturationLimit=-pi
  Integrator2 : Integrator  InitialCondition=[0;0;0;0;0;0]  UpperSaturationLimit=[170;135;166;190;120;360]*pi/180  LowerSaturationLimit=-[170;100;119;190;120;360]*pi/180
  the : Outport
  dthe : Outport  Port=2
  dt : Outport  Port=3
  ex : Outport  Port=4
  wires:
  Integrator2/1 -> Dynamics/4(the), the/1
  Dynamics/1(ddthe) -> Integrator/1
  Integrator/1 -> Dynamics/3(dthe), dthe/1, Integrator2/1
  to/1 -> Dynamics/1(t)
  Dynamics/2(dt) -> dt/1
  Fe/1 -> Dynamics/2(Fe)
  Dynamics/3(ex) -> ex/1
  [I] -> Dynamics/10(I)
  [Pic] -> Dynamics/9(Pic)
  [L] -> Dynamics/8(L)
  [m] -> Dynamics/7(m)
  Fv/1 -> Dynamics/5(Fv)
  Fc/1 -> Dynamics/6(Fc)

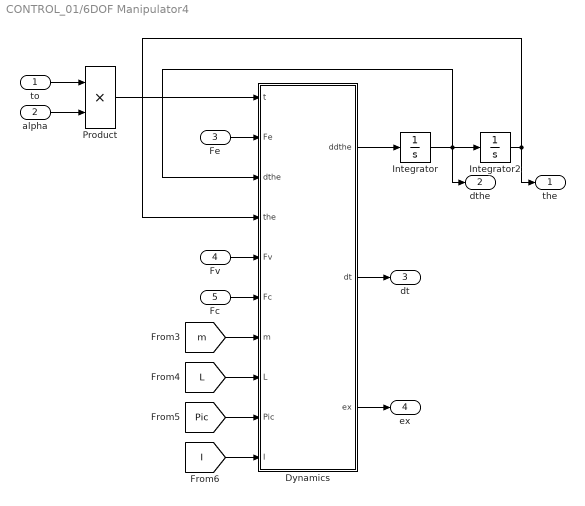
== system CONTROL_01/6DOF Manipulator4 ==
  to : Inport
  alpha : Inport  Port=2
  Fe : Inport  Port=3
  Fv : Inport  Port=4
  Fc : Inport  Port=5
  Dynamics : MATLAB Function  TreatAsAtomicUnit=on
  Integrator : Integrator  InitialCondition=[0;0;0;0;0;0]  UpperSaturationLimit=pi  LowerSaturationLimit=-pi
  Integrator2 : Integrator  InitialCondition=[0;0;0;0;0;0]  UpperSaturationLimit=[170;135;166;190;120;360]*pi/180  LowerSaturationLimit=-[170;100;119;190;120;360]*pi/180
  Product : Product
  the : Outport
  dthe : Outport  Port=2
  dt : Outport  Port=3
  ex : Outport  Port=4
  wires:
  Fc/1 -> Dynamics/6(Fc)
  Fv/1 -> Dynamics/5(Fv)
  [m] -> Dynamics/7(m)
  [L] -> Dynamics/8(L)
  [Pic] -> Dynamics/9(Pic)
  [I] -> Dynamics/10(I)
  Dynamics/3(ex) -> ex/1
  Fe/1 -> Dynamics/2(Fe)
  Dynamics/2(dt) -> dt/1
  Integrator/1 -> Integrator2/1, dthe/1, Dynamics/3(dthe)
  Dynamics/1(ddthe) -> Integrator/1
  Integrator2/1 -> the/1, Dynamics/4(the)
  to/1 -> Product/1
  Product/1 -> Dynamics/1(t)
  alpha/1 -> Product/2

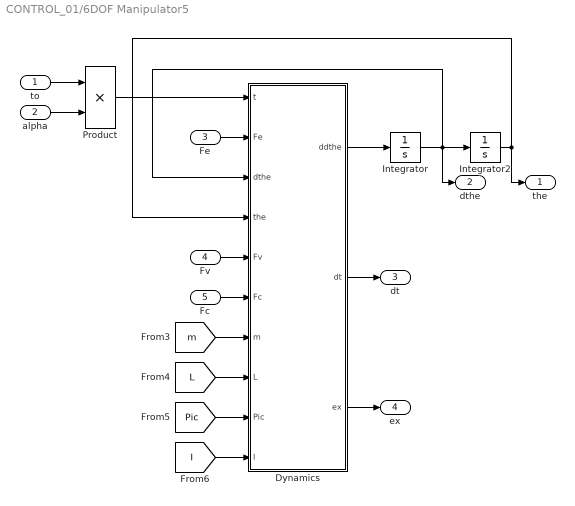
== system CONTROL_01/6DOF Manipulator5 ==
  to : Inport
  alpha : Inport  Port=2
  Fe : Inport  Port=3
  Fv : Inport  Port=4
  Fc : Inport  Port=5
  Dynamics : MATLAB Function  TreatAsAtomicUnit=on
  Integrator : Integrator  InitialCondition=[0;0;0;0;0;0]  UpperSaturationLimit=pi  LowerSaturationLimit=-pi
  Integrator2 : Integrator  InitialCondition=[0;0;0;0;0;0]  UpperSaturationLimit=[170;135;166;190;120;360]*pi/180  LowerSaturationLimit=-[170;100;119;190;120;360]*pi/180
  Product : Product
  the : Outport
  dthe : Outport  Port=2
  dt : Outport  Port=3
  ex : Outport  Port=4
  wires:
  Fc/1 -> Dynamics/6(Fc)
  Fv/1 -> Dynamics/5(Fv)
  [m] -> Dynamics/7(m)
  [L] -> Dynamics/8(L)
  [Pic] -> Dynamics/9(Pic)
  [I] -> Dynamics/10(I)
  Dynamics/3(ex) -> ex/1
  Fe/1 -> Dynamics/2(Fe)
  Dynamics/2(dt) -> dt/1
  Integrator/1 -> Integrator2/1, dthe/1, Dynamics/3(dthe)
  Dynamics/1(ddthe) -> Integrator/1
  Integrator2/1 -> the/1, Dynamics/4(the)
  alpha/1 -> Product/2
  to/1 -> Product/1
  Product/1 -> Dynamics/1(t)

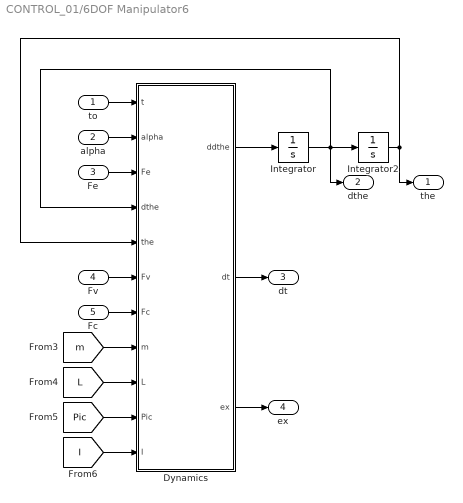
== system CONTROL_01/6DOF Manipulator6 ==
  to : Inport
  alpha : Inport  Port=2
  Fe : Inport  Port=3
  Fv : Inport  Port=4
  Fc : Inport  Port=5
  Dynamics : MATLAB Function  TreatAsAtomicUnit=on
  Integrator : Integrator  InitialCondition=[0;0;0;0;0;0]  UpperSaturationLimit=pi  LowerSaturationLimit=-pi
  Integrator2 : Integrator  InitialCondition=[0;0;0;0;0;0]  UpperSaturationLimit=[170;135;166;190;120;360]*pi/180  LowerSaturationLimit=-[170;100;119;190;120;360]*pi/180
  the : Outport
  dthe : Outport  Port=2
  dt : Outport  Port=3
  ex : Outport  Port=4
  wires:
  to/1 -> Dynamics/1(t)
  Integrator2/1 -> Dynamics/5(the), the/1
  Dynamics/1(ddthe) -> Integrator/1
  Integrator/1 -> Dynamics/4(dthe), dthe/1, Integrator2/1
  Dynamics/2(dt) -> dt/1
  Fe/1 -> Dynamics/3(Fe)
  Dynamics/3(ex) -> ex/1
  [I] -> Dynamics/11(I)
  [Pic] -> Dynamics/10(Pic)
  [L] -> Dynamics/9(L)
  [m] -> Dynamics/8(m)
  Fv/1 -> Dynamics/6(Fv)
  Fc/1 -> Dynamics/7(Fc)
  alpha/1 -> Dynamics/2(alpha)

== system CONTROL_01/PID Control ==
  the : Inport
  the_r : Inport  Port=2
  Kp : Inport  Port=3
  Ki : Inport  Port=4
  Kd : Inport  Port=5
  Derivative : Derivative
  Integrator : Integrator
  PID : MATLAB Function  TreatAsAtomicUnit=on
  Sum : Sum  Inputs=-+
  to : Outport
  wires:
  Sum/1 -> Derivative/1, Integrator/1, PID/1(e)
  the/1 -> Sum/1
  the_r/1 -> Sum/2
  Derivative/1 -> PID/3(ed)
  Integrator/1 -> PID/2(ei)
  Kp/1 -> PID/4(Kp)
  Ki/1 -> PID/5(Ki)
  Kd/1 -> PID/6(Kd)
  PID/1(to) -> to/1

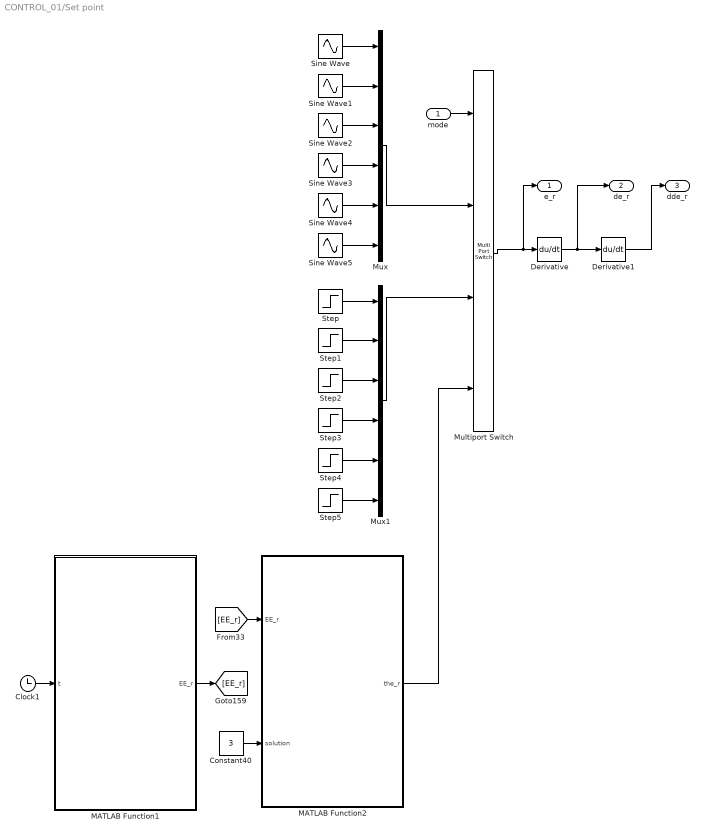
== system CONTROL_01/Set point ==
  mode : Inport
  Clock1 : Clock
  Constant40 : Constant  Value=3
  Derivative : Derivative
  Derivative1 : Derivative
  MATLAB Function1 : MATLAB Function  TreatAsAtomicUnit=on
  MATLAB Function2 : MATLAB Function  TreatAsAtomicUnit=on
  Multiport Switch : MultiPortSwitch
  Mux : Mux  Inputs=6
  Mux1 : Mux  Inputs=6
  Sine Wave{,1..5} (6 alike) : Sin  Amplitude=pi/6  Frequency=2*pi*0.1  SampleTime=0
  Step{,1..5} (6 alike) : Step  After=0  SampleTime=0
  e_r : Outport
  de_r : Outport  Port=2
  dde_r : Outport  Port=3
  wires:
  Sine Wave/1 -> Mux/1
  Sine Wave1/1 -> Mux/2
  Sine Wave2/1 -> Mux/3
  Sine Wave3/1 -> Mux/4
  Sine Wave4/1 -> Mux/5
  Sine Wave5/1 -> Mux/6
  Mux/1 -> Multiport Switch/2
  Mux1/1 -> Multiport Switch/3
  Step2/1 -> Mux1/3
  Step5/1 -> Mux1/6
  Step1/1 -> Mux1/2
  Step3/1 -> Mux1/4
  Step/1 -> Mux1/1
  Step4/1 -> Mux1/5
  Multiport Switch/1 -> e_r/1, Derivative/1
  Derivative/1 -> de_r/1, Derivative1/1
  Derivative1/1 -> dde_r/1
  mode/1 -> Multiport Switch/1
  [EE_r] -> MATLAB Function2/1(EE_r)
  Clock1/1 -> MATLAB Function1/1(t)
  MATLAB Function1/1(EE_r) -> [EE_r]
  Constant40/1 -> MATLAB Function2/2(solution)
  MATLAB Function2/1(the_r) -> Multiport Switch/4
